simulink model "rotation_d"  (R2020a)
settings: Solver=VariableStepAuto  StartTime=0.0  StopTime=10.0  RelTol=1e-3
values from neighbouring files (symbols this model uses):
  euler_angles_NfromB_0_deg = [0; 0; 0]    [p1partApartI.m]
  omega_BwrtN_rps = [0; 0; 0.11]    [p1partApartI.m]
libraries: coordinate_transforms x2, aerolibutil x1, sharedutil x1, sharedtransform x1
settings Model: Creator=Nikita  LastModifiedBy=Nikita

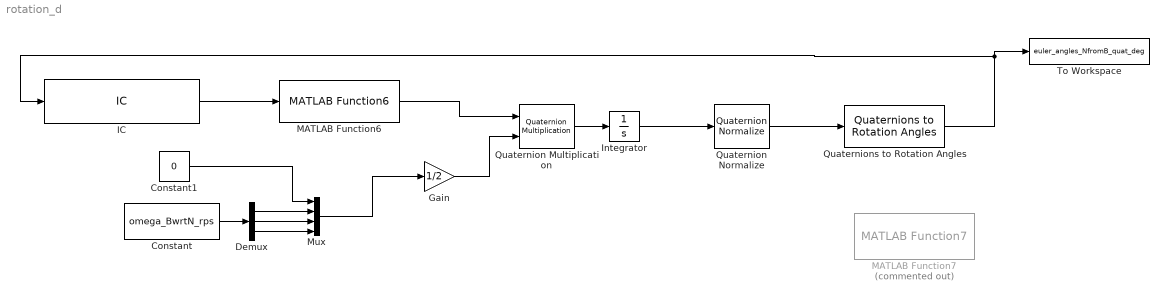
== system rotation_d ==
  Constant : Constant  Value=omega_BwrtN_rps
  Constant1 : Constant  Value=0
  Demux : Demux  Outputs=3
  Gain : Gain  Gain=1/2
  IC : InitialCondition  Value=euler_angles_NfromB_0_deg
  Integrator : Integrator
  MATLAB Function6 : coordinate_transforms/MATLAB Function6  SystemSampleTime=-1  Latency=0  AutoFrameSizeCalculation=off
  MATLAB Function7 : coordinate_transforms/MATLAB Function7  Commented=on  SystemSampleTime=-1  Latency=0  AutoFrameSizeCalculation=off
  Mux : Mux
  Quaternion Multiplication : aerolibutil/Quaternion Multiplication
  Quaternion Normalize : sharedutil/Quaternion Normalize  aMode=aMode
      settings: SourceProductBaseCode=AE,PW,MT,VE,VP
  Quaternions to Rotation Angles : sharedtransform/Quaternions to Rotation Angles  rotationOrder=ZYX  aMode=aMode
      settings: SourceProductBaseCode=AE,PW,MT,VE,VP
  To Workspace : ToWorkspace  VariableName=euler_angles_NfromB_quat_deg  SampleTime=-1
  wires:
  IC/1 -> MATLAB Function6/1
  MATLAB Function6/1 -> Quaternion Multiplication/1
  Gain/1 -> Quaternion Multiplication/2
  Quaternion Multiplication/1 -> Integrator/1
  Constant/1 -> Demux/1
  Demux/1 -> Mux/2
  Demux/2 -> Mux/3
  Demux/3 -> Mux/4
  Constant1/1 -> Mux/1
  Mux/1 -> Gain/1
  Integrator/1 -> Quaternion Normalize/1
  Quaternions to Rotation Angles/1 -> IC/1, To Workspace/1
  Quaternion Normalize/1 -> Quaternions to Rotation Angles/1
